simulink model "TST_HelloWorldModel"  (Simulink 7.4)
settings: Solver=FixedStepDiscrete  StartTime=0.0  StopTime=10.0  FixedStep=0.02  RelTol=1e-3
undefined symbols (not defined in the file): GBL_Constants_Feet2Meter, GBL_Definitions_EjectionCmd
settings Model: Creator=kharthforeign  LastModifiedBy=kharthforeign  BufferReuse=off
settings DataIOCC: SaveOutput=off  SignalLogging=off  SaveTime=off
settings OptimizationCC: BlockReduction=off  ConditionallyExecuteInputs=off  OptimizeBlockIOStorage=off  BufferReuse=off  ExpressionFolding=off  LocalBlockOutputs=off  InitFltsAndDblsToZero=on

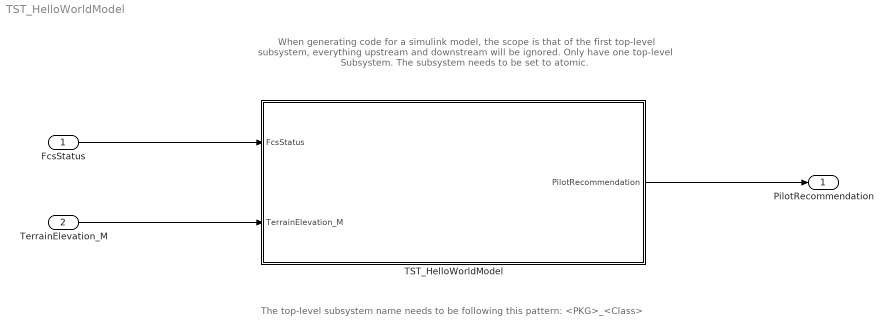
== system TST_HelloWorldModel ==
  note: When generating code for a simulink model, the scope is that of the first top-level subsystem,
      | everything upstream and downstream will be ignored.
      |
      | Only have one top-level Subsystem.
      | The subsystem needs to be set to atomic.
  note: The top-level subsystem name needs to be following this pattern:
      | <PKG>_<Class>
  FcsStatus : Inport  UseBusObject=on  OutDataType=fixdt(1, 16)  OutScaling=2^0
      settings: BusObject=FCS_FlightControlSystem_Status
  TerrainElevation_M : Inport  Port=2  PortDimensions=1  DataType=double  OutDataType=fixdt(1, 16)  OutScaling=2^0  OutDataTypeStr=double
  TST_HelloWorldModel : Subsystem  TreatAsAtomicUnit=on
  PilotRecommendation : Outport  PortDimensions=1  DataType=Specify via dialog  OutDataType=Enum: GBL_Definitions_EjectionCmd  OutDataTypeStr=Enum: GBL_Definitions_EjectionCmd
  wires:
  FcsStatus/1 -> TST_HelloWorldModel/1(FcsStatus)
  TerrainElevation_M/1 -> TST_HelloWorldModel/2(TerrainElevation_M)
  TST_HelloWorldModel/1(PilotRecommendation) -> PilotRecommendation/1

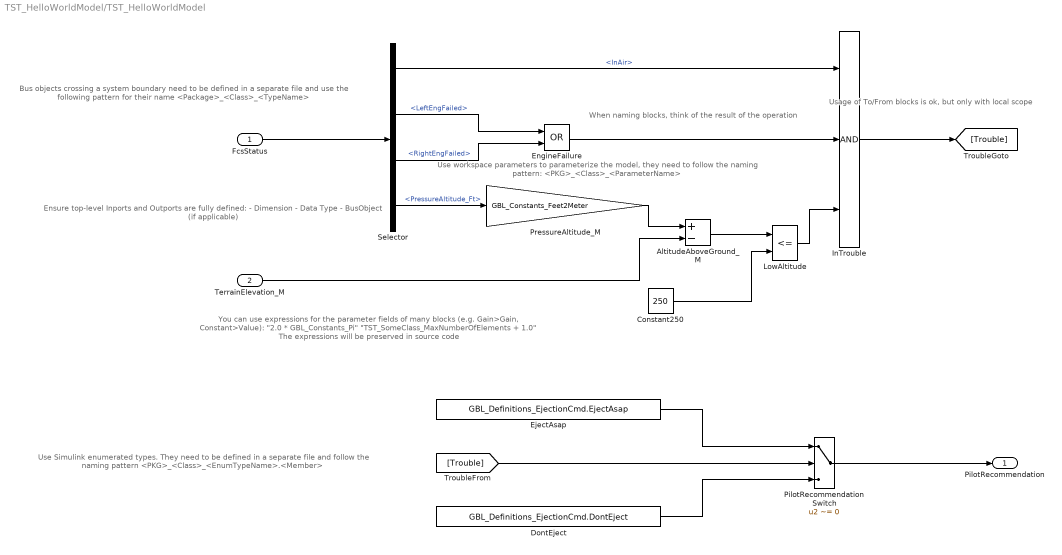
== system TST_HelloWorldModel/TST_HelloWorldModel ==
  note: Ensure top-level Inports and
      | Outports are fully defined:
      | - Dimension
      | - Data Type
      | - BusObject (if applicable)
  note: Usage of To/From blocks
      | is ok, but only with local scope
  note: When naming blocks, think of the
      | result of the operation
  note: Bus objects crossing a system
      | boundary need to be defined in a separate file
      | and use the following pattern for their name
      | <Package>_<Class>_<TypeName>
  note: Use workspace parameters to parameterize the model,
      | they need to follow the naming pattern:
      | <PKG>_<Class>_<ParameterName>
  note: You can use expressions for the parameter fields of many blocks
      | (e.g. Gain>Gain, Constant>Value):
      | "2.0 * GBL_Constants_Pi"
      | "TST_SomeClass_MaxNumberOfElements + 1.0"
      | The expressions will be preserved in source code
  note: Use Simulink enumerated types.
      | They need to be defined in a separate file
      | and follow the naming pattern
      | <PKG>_<Class>_<EnumTypeName>.<Member>
  FcsStatus : Inport  UseBusObject=on  OutDataType=fixdt(1, 16)  OutScaling=2^0
      settings: BusObject=FCS_FlightControlSystem_Status
  TerrainElevation_M : Inport  Port=2  PortDimensions=1  DataType=double  OutDataType=fixdt(1, 16)  OutScaling=2^0  OutDataTypeStr=double
  AltitudeAboveGround_M : Sum  Inputs=+-  OutDataType=fixdt(1, 16)  OutScaling=2^-10
  Constant250 : Constant  Value=250  OutDataTypeMode=double  OutDataType=fixdt(1, 16)  OutScaling=2^0  OutDataTypeStr=double
  DontEject : Constant  Value=GBL_Definitions_EjectionCmd.DontEject  OutDataTypeMode=Specify via dialog  OutDataType=Enum: GBL_Definitions_EjectionCmd  ConRadixGroup=Best Precision: Vector-wise  OutDataTypeStr=Enum: GBL_Definitions_EjectionCmd
  EjectAsap : Constant  Value=GBL_Definitions_EjectionCmd.EjectAsap  OutDataTypeMode=Specify via dialog  OutDataType=Enum: GBL_Definitions_EjectionCmd  ConRadixGroup=Best Precision: Vector-wise  OutDataTypeStr=Enum: GBL_Definitions_EjectionCmd
  EngineFailure : Logic  Operator=OR  AllPortsSameDT=off  OutDataTypeMode=boolean  LogicDataType=fixdt(0, 8)  OutDataTypeStr=boolean
  InTrouble : Logic  Inputs=3  AllPortsSameDT=off  OutDataTypeMode=boolean  LogicDataType=fixdt(0, 8)  OutDataTypeStr=boolean
  LowAltitude : RelationalOperator  Operator=<=  LogicOutDataTypeMode=boolean  LogicDataType=fixdt(0, 8)  OutDataTypeStr=boolean
  PilotRecommendationSwitch : Switch  Criteria=u2 ~= 0  OutDataTypeMode=Specify via dialog  OutDataType=Enum: GBL_Definitions_EjectionCmd  OutDataTypeStr=Enum: GBL_Definitions_EjectionCmd
  PressureAltitude_M : Gain  Gain=GBL_Constants_Feet2Meter  ParameterDataType=fixdt(1, 16)  ParameterScaling=2^0  OutDataType=fixdt(1, 16)  OutScaling=2^0
  Selector : BusSelector  OutputSignals=InAir,LeftEngFailed,RightEngFailed,PressureAltitude_Ft
  PilotRecommendation : Outport  PortDimensions=1  DataType=Specify via dialog  OutDataType=Enum: GBL_Definitions_EjectionCmd  OutDataTypeStr=Enum: GBL_Definitions_EjectionCmd
  wires:
  FcsStatus/1 -> Selector/1
  Selector/2 -> EngineFailure/1  "<LeftEngFailed>"
  Selector/3 -> EngineFailure/2  "<RightEngFailed>"
  Selector/4 -> PressureAltitude_M/1  "<PressureAltitude_Ft>"
  PressureAltitude_M/1 -> AltitudeAboveGround_M/1
  TerrainElevation_M/1 -> AltitudeAboveGround_M/2
  AltitudeAboveGround_M/1 -> LowAltitude/1
  Constant250/1 -> LowAltitude/2
  Selector/1 -> InTrouble/1  "<InAir>"
  EngineFailure/1 -> InTrouble/2
  LowAltitude/1 -> InTrouble/3
  [Trouble] -> PilotRecommendationSwitch/2
  PilotRecommendationSwitch/1 -> PilotRecommendation/1
  EjectAsap/1 -> PilotRecommendationSwitch/1
  DontEject/1 -> PilotRecommendationSwitch/3
  InTrouble/1 -> [Trouble]
